simulink model "Trajectory_Tracking_Car_FL_MPC"  (R2024b)
settings: Solver=FixedStepAuto  StartTime=0.0  StopTime=63  FixedStep=Ts  RelTol=1e-3
values from neighbouring files (symbols this model uses):
  alpha = 3    [Setup_Trajectory_FL_MPC.m]    (also in Setup_trajectory_Backstepping.m; Setup_trajectory_NL_MPC.m)
  beta = 1.7    [Setup_Trajectory_FL_MPC.m]    (also in Setup_trajectory_Backstepping.m; Setup_trajectory_NL_MPC.m)
  Delta = 0.35    [Setup_Trajectory_FL_MPC.m]    (also in Setup_trajectory_NL_MPC.m)
  g_N = P_N.b    [Setup_Trajectory_FL_MPC.m]
  H_N = P_N.A    [Setup_Trajectory_FL_MPC.m]
  H_w = H_w/g_w(1)    [Setup_Trajectory_FL_MPC.m]    (also in Setup_trajectory_NL_MPC.m)
  Linv = linsolve(L,eye(size(L)),struct('LT',true))    [Setup_Trajectory_FL_MPC.m]
  N = 10    [Setup_Trajectory_FL_MPC.m]    (also in Setup_trajectory_Backstepping.m; Setup_trajectory_NL_MPC.m = 5)
  q0 = [x0;y0;theta0;phi0]    [Setup_Trajectory_FL_MPC.m]    (also in Setup_trajectory_Backstepping.m; Setup_trajectory_NL_MPC.m)
  qu = 0.00001    (= 1e-05)    [Setup_Trajectory_FL_MPC.m]    (also in Setup_trajectory_NL_MPC.m = 0.0001)
  qz = 10    [Setup_Trajectory_FL_MPC.m]    (also in Setup_trajectory_NL_MPC.m = 1)
  thetar = unwrap(atan2(ydr./v1r,xdr./v1r))    [Setup_Trajectory_FL_MPC.m]    (also in Setup_trajectory_Backstepping.m; Setup_trajectory_NL_MPC.m)
  Ts = 0.01    [Setup_Trajectory_FL_MPC.m]    (also in Setup_trajectory_Backstepping.m; Setup_trajectory_NL_MPC.m = 0.1)
  v1max = 2    [Setup_Trajectory_FL_MPC.m]    (also in Setup_trajectory_Backstepping.m; Setup_trajectory_NL_MPC.m)
  v2max = 2    [Setup_Trajectory_FL_MPC.m]    (also in Setup_trajectory_Backstepping.m = 10; Setup_trajectory_NL_MPC.m)
settings Model: Creator=cricr  LastModifiedBy=tirio
settings SolverCC: AlgebraicLoopSolver=TrustRegion
settings DataIOCC: ReturnWorkspaceOutputs=off
settings OptimizationCC: ReuseModelBlockBuffer=off
settings DebuggingCC: UnconnectedInputMsg=warning  UnconnectedOutputMsg=warning  UnconnectedLineMsg=warning  ArithmeticOperatorsInVariantConditions=warning
settings ModelReferenceCC: EnableRefExpFcnMdlSchedulingChecks=on
settings SFSimCC: SimUseLocalCustomCode=off  CustomCodeUndefinedFunction=UseInterfaceOnly
settings RTWCC: RTWUseLocalCustomCode=off  GPUComputeCapability=3.5

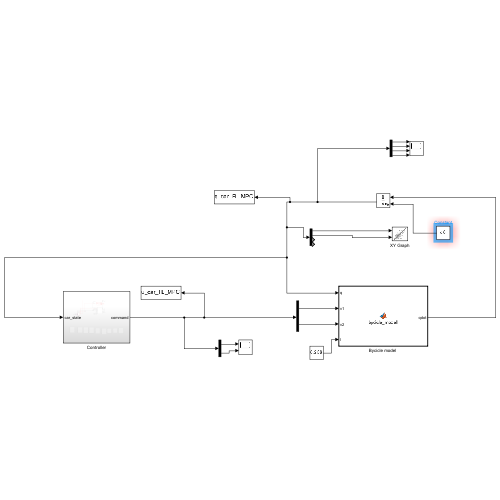
[thumbnail: Simulink's stored preview of the top-level diagram]
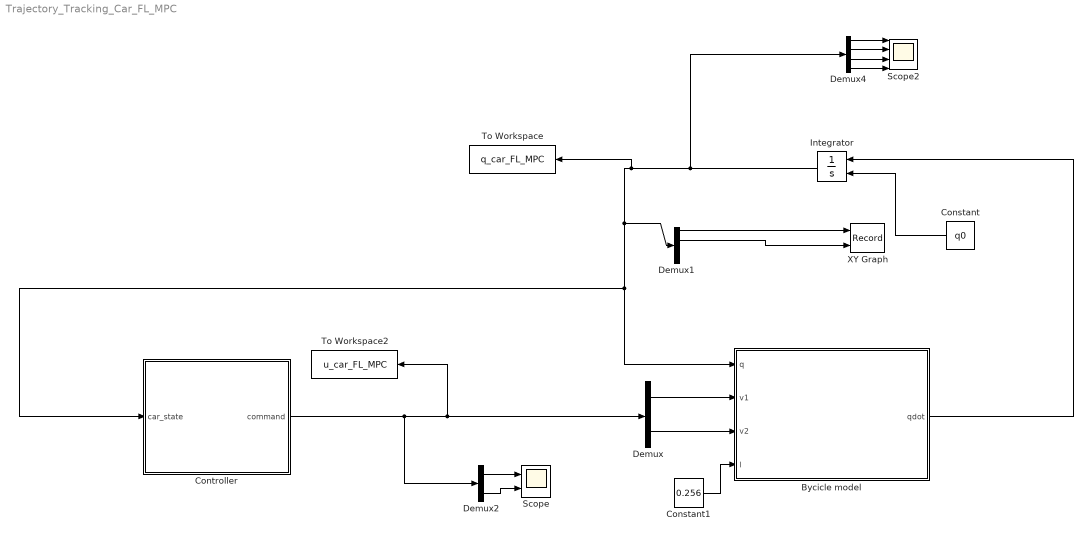
== system Trajectory_Tracking_Car_FL_MPC ==
  "Bycicle model " : MATLAB Function  TreatAsAtomicUnit=on
  Constant : Constant  Value=q0
  Constant1 : Constant  Value=0.256
  Controller : Subsystem
  Demux : Demux  Outputs=2
  Demux1 : Demux
  Demux2 : Demux  Outputs=2
  Demux4 : Demux
  Integrator : Integrator  InitialConditionSource=external
  Scope : Scope  NumInputPorts=2
  Scope2 : Scope  NumInputPorts=4
  To Workspace : ToWorkspace  VariableName=q_car_FL_MPC  SaveFormat=Timeseries  SampleTime=-1
  To Workspace2 : ToWorkspace  VariableName=u_car_FL_MPC  SaveFormat=Timeseries  SampleTime=-1
  XY Graph : Record  FileSettingsInternal="{\"entries\":[{\"content\":{\"excelSettings\":{\"content\":{},\"type\":\"Streamout.ExcelSettings\"}},\"type\":\"Streamout.FileSettingStorage\",\"uuid\":\"\"}],\"packageUris\":[\"http:\\/\\/schema.mathworks.com\\/mf0\\/streamout_blocks\\/R2020a\"],\"version\":\"1.0\"}"  Layout=[1 1]  SignalsInternal="{\"entries\":[{\"content\":{\"signals\":[{\"content\":{\"blockPath\":[],\"dimensions\":[1],\"domain\":\"\",\"lineColor\":\"#77ac30\",\"port\":1,\"signalID\":1,\"signalName\":\"Demux1:1\"},\"type\":\"RecordBlkView.Signal\",\"uuid\":\"\"},{\"content\":{\"blockPath\":[],\"dimensions\":[1],\"domain\":\"\",\"lineColor\":\"#4dbeee\",\"port\":2,\"signalID\":2,\"signalName\":\"Demux1:2\"},\"type\":\"RecordBlkView.Signal\",\"uuid\":\"\"}]},\"type\":\"RecordBlkView.InputSignals\",\"uuid\":\"\"}],\"packageUris\":[\"http:\\/\\/schema.mathworks.com\\/mf0\\/streamout_blocks\\/R2020a\"],\"version\":\"1.0\"}"  VisualizationBindings="{\"xyplotplugin\":{\"info\":[{\"series\":[],\"subplotID\":1}]}}"  CompatibilityTag=XY
  wires:
  "Bycicle model "/1(qdot) -> Integrator/1
  Constant1/1 -> "Bycicle model "/4(l)
  Demux/1 -> "Bycicle model "/2(v1)
  Demux/2 -> "Bycicle model "/3(v2)
  Demux1/1 -> XY Graph/1
  Demux1/2 -> XY Graph/2
  Demux4/4 -> Scope2/4
  Demux4/2 -> Scope2/2
  Demux4/3 -> Scope2/3
  Demux4/1 -> Scope2/1
  Constant/1 -> Integrator/2
  Integrator/1 -> Demux4/1, To Workspace/1, Controller/1(car_state), "Bycicle model "/1(q), Demux1/1
  Demux2/2 -> Scope/2
  Demux2/1 -> Scope/1
  Controller/1(command) -> Demux2/1, To Workspace2/1, Demux/1

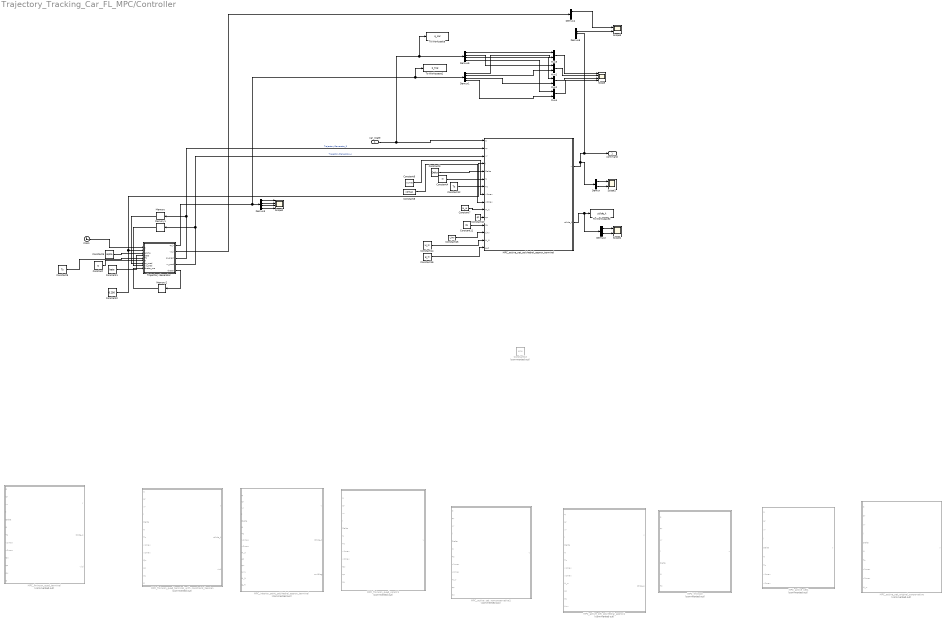
== system Trajectory_Tracking_Car_FL_MPC/Controller ==
  car_state : Inport
  Clock : Clock
  Constant : Constant  Value=N
  Constant1 : Constant  Value=beta
  Constant10 : Constant  Value=qz
  Constant11 : Constant  Value=qu
  Constant12 : Constant  Value=Ts
  Constant13 : Constant  Commented=on  Value=Linv
  Constant14 : Constant  Value=H_N
  Constant15 : Constant  Value=Linv
  Constant16 : Constant  Value=g_N
  Constant2 : Constant  Value=0.256
  Constant3 : Constant  Value=Delta
  Constant4 : Constant  Value=N
  Constant5 : Constant  Value=alpha
  Constant6 : Constant  Value=v1max
  Constant7 : Constant  Value=H_w
  Constant8 : Constant  Value=v2max
  Constant9 : Constant  Value=Ts
  Demux{,2,4,6} (4 alike) : Demux  Outputs=2
  Demux1 : Demux
  Demux3 : Demux
  Demux5 : Demux
  MPC_active_set1 : MATLAB Function  Commented=on  TreatAsAtomicUnit=on
  MPC_active_set_nonconservative1 : MATLAB Function  Commented=on  TreatAsAtomicUnit=on
  MPC_active_set_original_conservative : MATLAB Function  Commented=on  TreatAsAtomicUnit=on
  MPC_active_set_polyhedral_approx1 : MATLAB Function  Commented=on  TreatAsAtomicUnit=on
  MPC_active_set_polyhedral_approx_terminal : MATLAB Function  TreatAsAtomicUnit=on
  MPC_fmincon : MATLAB Function  Commented=on  TreatAsAtomicUnit=on
  MPC_fmincon_quad_constr1 : MATLAB Function  Commented=on  TreatAsAtomicUnit=on
  MPC_fmincon_quad_terminal : MATLAB Function  Commented=on  TreatAsAtomicUnit=on
  MPC_fmincon_quad_terminal_with_constraint_hessian : MATLAB Function  Commented=on  TreatAsAtomicUnit=on
  MPC_interior_point_polyhedral_approx_terminal : MATLAB Function  Commented=on  TreatAsAtomicUnit=on
  Memory : Memory  InitialCondition=zeros(4,N)
  Memory1 : Memory  InitialCondition=zeros(2,N)
  Memory2 : Memory  InitialCondition=thetar(1)
  Mux{1..4} (4 alike) : Mux  Inputs=2
  Scope : Scope  NumInputPorts=4
  Scope1 : Scope  NumInputPorts=2
  Scope2 : Scope  NumInputPorts=4
  Scope3 : Scope  NumInputPorts=2
  Scope4 : Scope  NumInputPorts=2
  To Workspace : ToWorkspace  VariableName=q_car  SaveFormat=Timeseries  SampleTime=-1
  To Workspace1 : ToWorkspace  VariableName=q_traj  SaveFormat=Timeseries  SampleTime=-1
  To Workspace2 : ToWorkspace  VariableName=ztilde_k  SaveFormat=Timeseries  SampleTime=-1
  Trajectory Generator : MATLAB Function  TreatAsAtomicUnit=on
  command : Outport
  wires:
  Demux5/2 -> Mux1/1
  Constant6/1 -> MPC_active_set_polyhedral_approx_terminal/8(v1max)
  Demux6/1 -> Scope3/2
  Demux5/4 -> Mux4/1
  Mux2/1 -> Scope/3
  Mux3/1 -> Scope/1
  Demux3/1 -> Scope2/1
  Demux4/1 -> Scope3/1
  Demux1/3 -> Mux2/2
  Mux1/1 -> Scope/2
  Demux1/4 -> Mux4/2
  Mux4/1 -> Scope/4
  Constant7/1 -> MPC_active_set_polyhedral_approx_terminal/10(H_w)
  Demux3/2 -> Scope2/2
  Demux5/1 -> Mux3/1
  Demux3/4 -> Scope2/4
  car_state/1 -> To Workspace/1, Demux5/1, MPC_active_set_polyhedral_approx_terminal/1(q)
  Constant8/1 -> MPC_active_set_polyhedral_approx_terminal/9(v2max)
  Demux1/1 -> Mux3/2
  MPC_active_set_polyhedral_approx_terminal/1(v) -> Demux/1, Demux6/1, command/1
  Demux1/2 -> Mux1/2
  Demux5/3 -> Mux2/1
  Demux3/3 -> Scope2/3
  Memory1/1 -> Trajectory Generator/8("vr_pred ")
  Memory/1 -> Trajectory Generator/7("qr_pred ")
  Trajectory Generator/3(qr_pred) -> MPC_active_set_polyhedral_approx_terminal/2(qr), Memory/1  "TrajectoryGenerator_3"
  Constant/1 -> Trajectory Generator/6(N)
  Trajectory Generator/4(vr_pred) -> MPC_active_set_polyhedral_approx_terminal/3(vr), Memory1/1  "TrajectoryGenerator_4"
  Constant1/1 -> Trajectory Generator/4(beta)
  Constant2/1 -> MPC_active_set_polyhedral_approx_terminal/4(l), Trajectory Generator/2(l)
  Constant9/1 -> Trajectory Generator/5(Ts)
  Constant5/1 -> Trajectory Generator/3(alpha)
  Trajectory Generator/5(thetar) -> Memory2/1
  Clock/1 -> Trajectory Generator/1(t)
  Memory2/1 -> Trajectory Generator/9(thetar_pre)
  Trajectory Generator/2(vr_k) -> Demux4/1
  Trajectory Generator/1(qr_k) -> To Workspace1/1, Demux1/1, Demux3/1
  Constant11/1 -> MPC_active_set_polyhedral_approx_terminal/12(qu)
  Constant3/1 -> MPC_active_set_polyhedral_approx_terminal/5(Delta)
  Constant12/1 -> MPC_active_set_polyhedral_approx_terminal/7(Ts)
  Constant14/1 -> MPC_active_set_polyhedral_approx_terminal/14(H_N)
  Demux/1 -> Scope1/1
  Demux/2 -> Scope1/2
  Constant15/1 -> MPC_active_set_polyhedral_approx_terminal/13(Linv)
  Demux2/2 -> Scope4/2
  Demux2/1 -> Scope4/1
  MPC_active_set_polyhedral_approx_terminal/2(ztilde_k) -> Demux2/1, To Workspace2/1
  Constant16/1 -> MPC_active_set_polyhedral_approx_terminal/15(g_N)
  Constant4/1 -> MPC_active_set_polyhedral_approx_terminal/6(N)
  Constant10/1 -> MPC_active_set_polyhedral_approx_terminal/11(qz)

== matlab function Trajectory_Tracking_Car_FL_MPC/Controller/Trajectory Generator ==
  data: t input; qr_k output; vr_k output; l input; alpha input; beta input; Ts input; qr_pred output size=[4 N]; vr_pred output size=[2 N]; N input; qr_pred input; vr_pred input; thetar_pre input; thetar output
function [qr_k,vr_k,qr_pred, vr_pred,thetar] = Trajectory(t,l,alpha,beta,Ts,N,qr_pred,vr_pred,thetar_pre)




xr=alpha*sin(t/beta);
yr=alpha*sin(t/(2*beta));

xdr=alpha*cos(t/beta)*(1/(beta));
ydr=alpha*cos(t/(2*beta))*(1/(2*beta));


xddr=-alpha*sin(t/beta)*(1/(beta))^2;
yddr=-alpha*sin(t/(2*beta))*(1/(2*beta))^2;

xdddr=-alpha*cos(t/beta)*(1/(beta))^3;
ydddr=-alpha*cos(t/(2*beta))*(1/(2*beta))^3;

%Driving velocity reference
v1r=sqrt(xdr^2+ydr^2); %Linear velocity of the trajectory


thetar=atan2(ydr/v1r,xdr/v1r);

theta=[thetar_pre thetar];

theta=unwrap(theta);
thetar=theta(2);


%Steering angle reference
phir=atan(l*(yddr*xdr-xddr*ydr)/v1r^3);

%Steering velocity reference
v2r=l*v1r*((ydddr*xdr-xdddr*ydr)*v1r^2-3*(yddr*xdr-xddr*ydr)*(xdr*xddr+ydr*yddr))/(v1r^6+l^2*(yddr*xdr-xddr*ydr)^2);


qr_k=[xr;yr;thetar;phir];
vr_k=[v1r;v2r];


for i=1:N
    t=t+(i-1)*Ts;
    xr=alpha*sin(t/beta);
    yr=alpha*sin(t/(2*beta));

    xdr=alpha*cos(t/beta)*(1/(beta));
    ydr=alpha*cos(t/(2*beta))*(1/(2*beta));


    xddr=-alpha*sin(t/beta)*(1/(beta))^2;
    yddr=-alpha*sin(t/(2*beta))*(1/(2*beta))^2;

    xdddr=-alpha*cos(t/beta)*(1/(beta))^3;
    ydddr=-alpha*cos(t/(2*beta))*(1/(2*beta))^3;



    %Driving velocity reference
    v1r=sqrt(xdr^2+ydr^2); %Linear velocity of the trajectory

    

    thetar=atan2(ydr/v1r,xdr/v1r);

    if i==1
        theta=[thetar_pre thetar];
        theta=unwrap(theta);
        thetar=theta(2);
        thetar_pre=thetar;

    else
       
        theta=[thetar_pre thetar];
        theta=unwrap(theta);
        thetar=theta(2);


    end


    %Steering angle reference
    phir=atan(l*(yddr*xdr-xddr*ydr)/v1r^3);

    %Steering velocity reference
    v2r=l*v1r*((ydddr*xdr-xdddr*ydr)*v1r^2-3*(yddr*xdr-xddr*ydr)*(xdr*xddr+ydr*yddr))/(v1r^6+l^2*(yddr*xdr-xddr*ydr)^2);



    %Nonlinear model reference state
    qr_pred(:,i)=[xr;yr;thetar;phir];
    vr_pred(:,i)=[v1r;v2r];

end

 qr_pred(3,:)= unwrap(qr_pred(3,:));

== matlab function Trajectory_Tracking_Car_FL_MPC/Controller/MPC_active_set_nonconservative1 ==
  data: q input; v output; qr input; vr input; l input; Delta input; N input; Ts input; v1max input; v2max input; H_w input; qz input; qu input
function v = MPC_analytical(q,qr,vr,l,Delta,N,Ts,v1max,v2max,H_w,qz,qu)


x=q(1); y=q(2); theta=q(3); phi=q(4);

%Feedback linearized system state
z_k=[x+l*cos(theta)+Delta*cos(phi+theta);
    y+l*sin(theta)+Delta*sin(phi+theta)];


Wr=zeros(2*N,1);
R=zeros(2*N,1);



for i=1:N
    xr=qr(1,i); yr=qr(2,i); thetar=qr(3,i); phir=qr(4,i);
    v1r=vr(1,i); v2r=vr(2,i);

    %Feedback linearized system reference at time k+i
    zr_k=[xr+l*cos(thetar)+Delta*cos(phir+thetar);
        yr+l*sin(thetar)+Delta*sin(phir+thetar)];

    R(2*i-1:2*i,1)=zr_k;

    %Feedback Linearization reference transformation
    T_FL_r=[cos(thetar)-tan(phir)*(sin(thetar)+Delta*sin(thetar+phir)/l) -Delta*sin(thetar+phir);
        sin(thetar)+tan(phir)*(cos(thetar)+Delta*cos(thetar+phir)/l) Delta*cos(thetar+phir)];

    ur_k=T_FL_r*[v1r;v2r];

    Wr(2*i-1:2*i,1)=ur_k;


end


%Feedback Linearization state transformation
T_FL=[cos(theta)-tan(phi)*(sin(theta)+Delta*sin(theta+phi)/l) -Delta*sin(theta+phi);
    sin(theta)+tan(phi)*(cos(theta)+Delta*cos(theta+phi)/l) Delta*cos(theta+phi)];





Phi=repmat(eye(2),N,1);
Theta=Ts*repmat(eye(2),N);
Theta=tril(Theta);
Qhat=qz*eye(2*N);
Rhat=qu*eye(2*N);







H_obj=Theta'*Qhat*Theta+Rhat;
f_obj=Theta'*Qhat*Phi*z_k-Theta'*Qhat*Theta*Wr-Theta'*Qhat*R;
% 
% T=[-1 0; 0 -1; 1 0; 0 1];
% Hk=T/T_FL;
% g=[v1max;v2max;v1max;v2max];
% 
% H_constr=zeros(4,2*N);
% H_constr(1:4,1:2)=Hk;

% for i=1:N-1
%     
%     H_constr(4+(i-1)*Nc+1:4+(i-1)*Nc+Nc,2*i+1:2*i+2)=H_w;
% 
% 
% end


% 
% g_constr=zeros(size(H_constr,1),1);
% g_constr(1:4)=g;
% 
% 
% 

% options = optimoptions('quadprog','Algorithm','active-set');
% usol =  quadprog(H_obj,f_obj,H_constr,g_constr,[],[],[],[],zeros(2*N,1),options);




% opt.MaxIterations = 100;
% opt.ConstraintTolerance = 1.0e-6;
% % opt.OptimalityTolerance = 1.0e-6;
% 
% opt = mpcInteriorPointOptions;
% usol=mpcInteriorPointSolver(H_obj,f_obj,H_constr,g_constr,zeros(0,2*N),zeros(0,1),zeros(2*N,1),opt);
% % 

% opt.UseHessianAsInput = true;
% iA0 = false(size(g_constr));
% usol=mpcActiveSetSolver(H_obj,f_obj,H_constr,g_constr,zeros(0,2*N),zeros(0,1),iA0,opt);



usol=-H_obj\f_obj;

uk=usol(1:2);



v=T_FL\uk;

== matlab function Trajectory_Tracking_Car_FL_MPC/Controller/MPC_active_set_polyhedral_approx_terminal ==
  data: q input; v output; qr input; vr input; l input; Delta input; N input; Ts input; v1max input; v2max input; H_w input; qz input; qu input; Linv input; H_N input; ztilde_k output; g_N input
function [v,ztilde_k] = MPC_active_set_polyhedral_approx(q,qr,vr,l,Delta,N,Ts,v1max,v2max,H_w,qz,qu,Linv,H_N,g_N)


x=q(1); y=q(2); theta=q(3); phi=q(4);

%Feedback linearized system state
z_k=[x+l*cos(theta)+Delta*cos(phi+theta);
     y+l*sin(theta)+Delta*sin(phi+theta)];


xr=qr(1,1); yr=qr(2,1); thetar=qr(3,1); phir=qr(4,1);
%Feedback linearized system reference at time k+i
zr_k=[xr+l*cos(thetar)+Delta*cos(phir+thetar);
      yr+l*sin(thetar)+Delta*sin(phir+thetar)];

ztilde_k=z_k-zr_k;


Wr=zeros(2*N,1);
% R=zeros(2*N,1);



for i=1:N
    thetar=qr(3,i); phir=qr(4,i);
    v1r=vr(1,i); v2r=vr(2,i);

    %     R(2*i-1:2*i,1)=zr_k;

    %Feedback Linearization reference transformation
    T_FL_r=[cos(thetar)-tan(phir)*(sin(thetar)+Delta*sin(thetar+phir)/l) -Delta*sin(thetar+phir);
        sin(thetar)+tan(phir)*(cos(thetar)+Delta*cos(thetar+phir)/l) Delta*cos(thetar+phir)];

    ur_k=T_FL_r*[v1r;v2r];

    Wr(2*i-1:2*i,1)=ur_k;


end


%Feedback Linearization state transformation
T_FL=[cos(theta)-tan(phi)*(sin(theta)+Delta*sin(theta+phi)/l) -Delta*sin(theta+phi);
    sin(theta)+tan(phi)*(cos(theta)+Delta*cos(theta+phi)/l) Delta*cos(theta+phi)];





Phi=repmat(eye(2),N,1);
Theta=Ts*repmat(eye(2),N);
Theta=tril(Theta);
Qhat=qz*eye(2*N);
Rhat=qu*eye(2*N);
Theta_N=Theta(2*N-1:2*N,:);
Phi_N=eye(2);


% H_obj=Theta'*Qhat*Theta+Rhat;
f_obj=Theta'*Qhat*Phi*ztilde_k-Theta'*Qhat*Theta*Wr-Rhat*Wr;

T=[-1 0; 0 -1; 1 0; 0 1];
Hk=T/T_FL;
g=[v1max;v2max;v1max;v2max];



Nc1=size(H_w,1);
H_constr1=zeros(4+Nc1*(N-1),2*N);
H_constr1(1:4,1:2)=Hk;

for i=1:N-1
    
    H_constr1(4+(i-1)*Nc1+1:4+(i-1)*Nc1+Nc1,2*i+1:2*i+2)=H_w;


end

g_constr1=ones(size(H_constr1,1),1);
g_constr1(1:4)=g;



H_constr2=H_N*Theta_N;
g_constr2=g_N-H_N*Phi_N*ztilde_k;

H_constr=[H_constr1;H_constr2];
g_constr=[g_constr1;g_constr2];


% options = optimoptions('quadprog','Algorithm','active-set');
% usol =  quadprog(H_obj,f_obj,H_constr,g_constr,[],[],[],[],zeros(2*N,1),options);




% opt = mpcInteriorPointOptions;
% 
% opt.MaxIterations = 100;
% opt.ConstraintTolerance = 1.0e-6;
% opt.OptimalityTolerance = 1.0e-6;
% 
% usol=mpcInteriorPointSolver(H_obj,f_obj,H_constr,g_constr,zeros(0,2*N),zeros(0,1),zeros(2*N,1),opt);

%
opt = mpcActiveSetOptions;
% opt.UseHessianAsInput = true;
opt.UseHessianAsInput = false;
opt.MaxIterations = 50;
opt.ConstraintTolerance = 1.0e-6;
opt.OptimalityTolerance = 1.0e-6;

iA0 = false(size(g_constr));
% usol=mpcActiveSetSolver(H_obj,f_obj,H_constr,g_constr,zeros(0,2*N),zeros(0,1),iA0,opt);
usol=mpcActiveSetSolver(Linv,f_obj,H_constr,g_constr,zeros(0,2*N),zeros(0,1),iA0,opt);


check=H_constr2*usol<=g_constr2;
viol=true;
for i=1:length(check)
    viol=viol&check(i);
end

viol



disp('Next step')
uk=usol(1:2);



v=T_FL\uk;

== matlab function Trajectory_Tracking_Car_FL_MPC/Controller/MPC_active_set_polyhedral_approx1 ==
  data: q input; v output; qr input; vr input; l input; Delta input; N input; Ts input; v1max input; v2max input; H_w input; qz input; qu input; Linv input; ztilde_k output
function [v,ztilde_k]= MPC_active_set_polyhedral_approx(q,qr,vr,l,Delta,N,Ts,v1max,v2max,H_w,qz,qu,Linv)


x=q(1); y=q(2); theta=q(3); phi=q(4);

%Feedback linearized system state
z_k=[x+l*cos(theta)+Delta*cos(phi+theta);
     y+l*sin(theta)+Delta*sin(phi+theta)];


xr=qr(1,1); yr=qr(2,1); thetar=qr(3,1); phir=qr(4,1);
%Feedback linearized system reference at time k+i
zr_k=[xr+l*cos(thetar)+Delta*cos(phir+thetar);
      yr+l*sin(thetar)+Delta*sin(phir+thetar)];

ztilde_k=z_k-zr_k;


Wr=zeros(2*N,1);
% R=zeros(2*N,1);



for i=1:N
    thetar=qr(3,i); phir=qr(4,i);
    v1r=vr(1,i); v2r=vr(2,i);

    %     R(2*i-1:2*i,1)=zr_k;

    %Feedback Linearization reference transformation
    T_FL_r=[cos(thetar)-tan(phir)*(sin(thetar)+Delta*sin(thetar+phir)/l) -Delta*sin(thetar+phir);
        sin(thetar)+tan(phir)*(cos(thetar)+Delta*cos(thetar+phir)/l) Delta*cos(thetar+phir)];

    ur_k=T_FL_r*[v1r;v2r];

    Wr(2*i-1:2*i,1)=ur_k;


end


%Feedback Linearization state transformation
T_FL=[cos(theta)-tan(phi)*(sin(theta)+Delta*sin(theta+phi)/l) -Delta*sin(theta+phi);
    sin(theta)+tan(phi)*(cos(theta)+Delta*cos(theta+phi)/l) Delta*cos(theta+phi)];





Phi=repmat(eye(2),N,1);
Theta=Ts*repmat(eye(2),N);
Theta=tril(Theta);
Qhat=qz*eye(2*N);
Rhat=qu*eye(2*N);


% H_obj=Theta'*Qhat*Theta+Rhat;
f_obj=Theta'*Qhat*Phi*ztilde_k-Theta'*Qhat*Theta*Wr-Rhat*Wr;

T=[-1 0; 0 -1; 1 0; 0 1];
Hk=T/T_FL;
g=[v1max;v2max;v1max;v2max];



Nc=size(H_w,1);
H_constr=zeros(4+Nc*(N-1),2*N);
H_constr(1:4,1:2)=Hk;

for i=1:N-1
    
    H_constr(4+(i-1)*Nc+1:4+(i-1)*Nc+Nc,2*i+1:2*i+2)=H_w;


end

g_constr=ones(size(H_constr,1),1);
g_constr(1:4)=g;





% options = optimoptions('quadprog','Algorithm','active-set');
% usol =  quadprog(H_obj,f_obj,H_constr,g_constr,[],[],[],[],zeros(2*N,1),options);




% opt = mpcInteriorPointOptions;
% 
% opt.MaxIterations = 100;
% opt.ConstraintTolerance = 1.0e-6;
% opt.OptimalityTolerance = 1.0e-6;
% 
% usol=mpcInteriorPointSolver(H_obj,f_obj,H_constr,g_constr,zeros(0,2*N),zeros(0,1),zeros(2*N,1),opt);

%
opt = mpcActiveSetOptions;
% opt.UseHessianAsInput = true;
opt.UseHessianAsInput = false;
opt.MaxIterations = 50;
opt.ConstraintTolerance = 1.0e-6;
opt.OptimalityTolerance = 1.0e-6;

iA0 = false(size(g_constr));
% usol=mpcActiveSetSolver(H_obj,f_obj,H_constr,g_constr,zeros(0,2*N),zeros(0,1),iA0,opt);
usol=mpcActiveSetSolver(Linv,f_obj,H_constr,g_constr,zeros(0,2*N),zeros(0,1),iA0,opt);

uk=usol(1:2);



v=T_FL\uk;

== matlab function Trajectory_Tracking_Car_FL_MPC/Controller/MPC_interior_point_polyhedral_approx_terminal ==
  data: q input; v output; qr input; vr input; l input; Delta input; N input; Ts input; v1max input; v2max input; H_w input; qz input; qu input; Linv input; H_N input; ztilde_k output; g_N input; exitflag output
function [v,ztilde_k,exitflag] = MPC_interior_point_polyhedral_approx(q,qr,vr,l,Delta,N,Ts,v1max,v2max,H_w,qz,qu,Linv,H_N,g_N)


x=q(1); y=q(2); theta=q(3); phi=q(4);

%Feedback linearized system state
z_k=[x+l*cos(theta)+Delta*cos(phi+theta);
     y+l*sin(theta)+Delta*sin(phi+theta)];


xr=qr(1,1); yr=qr(2,1); thetar=qr(3,1); phir=qr(4,1);
%Feedback linearized system reference at time k+i
zr_k=[xr+l*cos(thetar)+Delta*cos(phir+thetar);
      yr+l*sin(thetar)+Delta*sin(phir+thetar)];

ztilde_k=z_k-zr_k;


Wr=zeros(2*N,1);
% R=zeros(2*N,1);



for i=1:N
    thetar=qr(3,i); phir=qr(4,i);
    v1r=vr(1,i); v2r=vr(2,i);

    %     R(2*i-1:2*i,1)=zr_k;

    %Feedback Linearization reference transformation
    T_FL_r=[cos(thetar)-tan(phir)*(sin(thetar)+Delta*sin(thetar+phir)/l) -Delta*sin(thetar+phir);
        sin(thetar)+tan(phir)*(cos(thetar)+Delta*cos(thetar+phir)/l) Delta*cos(thetar+phir)];

    ur_k=T_FL_r*[v1r;v2r];

    Wr(2*i-1:2*i,1)=ur_k;


end


%Feedback Linearization state transformation
T_FL=[cos(theta)-tan(phi)*(sin(theta)+Delta*sin(theta+phi)/l) -Delta*sin(theta+phi);
    sin(theta)+tan(phi)*(cos(theta)+Delta*cos(theta+phi)/l) Delta*cos(theta+phi)];





Phi=repmat(eye(2),N,1);
Theta=Ts*repmat(eye(2),N);
Theta=tril(Theta);
Qhat=qz*eye(2*N);
Rhat=qu*eye(2*N);
Theta_N=Theta(2*N-1:2*N,:);
Phi_N=eye(2);


H_obj=Theta'*Qhat*Theta+Rhat;
f_obj=Theta'*Qhat*Phi*ztilde_k-Theta'*Qhat*Theta*Wr-Rhat*Wr;

T=[-1 0; 0 -1; 1 0; 0 1];
Hk=T/T_FL;
g=[v1max;v2max;v1max;v2max];



Nc1=size(H_w,1);
H_constr1=zeros(4+Nc1*(N-1),2*N);
H_constr1(1:4,1:2)=Hk;

for i=1:N-1
    
    H_constr1(4+(i-1)*Nc1+1:4+(i-1)*Nc1+Nc1,2*i+1:2*i+2)=H_w;


end

g_constr1=ones(size(H_constr1,1),1);
g_constr1(1:4)=g;



H_constr2=H_N*Theta_N;
g_constr2=g_N-H_N*Phi_N*ztilde_k;

H_constr=[H_constr1;H_constr2];
g_constr=[g_constr1;g_constr2];


% options = optimoptions('quadprog','Algorithm','active-set');
% usol =  quadprog(H_obj,f_obj,H_constr,g_constr,[],[],[],[],zeros(2*N,1),options);




opt = mpcInteriorPointOptions;

opt.MaxIterations = 100;
opt.ConstraintTolerance = 1.0e-6;
opt.OptimalityTolerance = 1.0e-6;

[usol, exitflag ]=mpcInteriorPointSolver(H_obj,f_obj,H_constr,g_constr,zeros(0,2*N),zeros(0,1),zeros(2*N,1),opt);

% %
% opt = mpcActiveSetOptions;
% % opt.UseHessianAsInput = true;
% opt.UseHessianAsInput = false;
% opt.MaxIterations = 50;
% opt.ConstraintTolerance = 1.0e-6;
% opt.OptimalityTolerance = 1.0e-6;
% 
% iA0 = false(size(g_constr));
% % usol=mpcActiveSetSolver(H_obj,f_obj,H_constr,g_constr,zeros(0,2*N),zeros(0,1),iA0,opt);
% usol=mpcActiveSetSolver(Linv,f_obj,H_constr,g_constr,zeros(0,2*N),zeros(0,1),iA0,opt);


check=H_constr*usol<=g_constr;
viol=true;
for i=1:length(check)
    viol=viol&check(i);
end

viol



disp('Next step')
uk=usol(1:2);



v=T_FL\uk;

== matlab function Trajectory_Tracking_Car_FL_MPC/Controller/MPC_fmincon_quad_constr1 ==
  data: q input; v output; qr input; vr input; l input; Delta input; N input; Ts input; v1max input; v2max input; Qu input; qz input; qu input
function v = MPC_quad_constr(q,qr,vr,l,Delta,N,Ts,v1max,v2max,Qu,qz,qu)


x=q(1); y=q(2); theta=q(3); phi=q(4);

%Feedback linearized system state
z_k=[x+l*cos(theta)+Delta*cos(phi+theta);
    y+l*sin(theta)+Delta*sin(phi+theta)];



xr=qr(1,1); yr=qr(2,1); thetar=qr(3,1); phir=qr(4,1);
%Feedback linearized system reference at time k+i
zr_k=[xr+l*cos(thetar)+Delta*cos(phir+thetar);
      yr+l*sin(thetar)+Delta*sin(phir+thetar)];

ztilde_k=z_k-zr_k;

Wr=zeros(2*N,1);


for i=1:N
    thetar=qr(3,i); phir=qr(4,i);
    v1r=vr(1,i); v2r=vr(2,i);

    %     R(2*i-1:2*i,1)=zr_k;

    %Feedback Linearization reference transformation
    T_FL_r=[cos(thetar)-tan(phir)*(sin(thetar)+Delta*sin(thetar+phir)/l) -Delta*sin(thetar+phir);
        sin(thetar)+tan(phir)*(cos(thetar)+Delta*cos(thetar+phir)/l) Delta*cos(thetar+phir)];

    ur_k=T_FL_r*[v1r;v2r];

    Wr(2*i-1:2*i,1)=ur_k;
end


%Feedback Linearization state transformation
T_FL=[cos(theta)-tan(phi)*(sin(theta)+Delta*sin(theta+phi)/l) -Delta*sin(theta+phi);
    sin(theta)+tan(phi)*(cos(theta)+Delta*cos(theta+phi)/l) Delta*cos(theta+phi)];





Phi=repmat(eye(2),N,1);
Theta=Ts*repmat(eye(2),N);
Theta=tril(Theta);
Qhat=qz*eye(2*N);
Rhat=qu*eye(2*N);




H_obj=Theta'*Qhat*Theta+Rhat;
f_obj=Theta'*Qhat*Phi*ztilde_k-Theta'*Qhat*Theta*Wr-Rhat*Wr;

T=[-1 0; 0 -1; 1 0; 0 1];
Hk=T/T_FL;
g=[v1max;v2max;v1max;v2max];











%obj_fun=@(W)(Phi*z_k+Theta*(W-Wr)-R)'*Qhat*(Phi*z_k+Theta*(W-Wr)-R)+W'*Rhat*W;

obj_fun=@(u)(u'*H_obj*u+f_obj'*u);

    function [c,ceq]=quad_constr(u,Hk,g,Qu,N)
        H_constr=zeros(4,2*N);
        H_constr(1:4,1:2)=Hk;

        g_constr=zeros(size(H_constr,1),1);
        g_constr(1:4)=g;

        c1=H_constr*u-g_constr;

        q_u=Qu(1,1);
        Qu_hat=zeros(2*N,2*N);

        for k=3:2*N
           Qu_hat(k,k)=q_u;
        end

        c2=u'*Qu_hat*u-1;

        

        c=[c1;c2];
        ceq=[];
    end



options=optimoptions('fmincon','Display','off','Algorithm','sqp');
usol = fmincon(obj_fun,zeros(N*2,1),[],[],[],[],[],[],@(u)quad_constr(u,Hk,g,Qu,N),options);



uk=usol(1:2);



v=T_FL\uk;


end

== matlab function Trajectory_Tracking_Car_FL_MPC/Controller/MPC_fmincon_quad_terminal ==
  data: q input; v output; qr input; vr input; l input; Delta input; N input; Ts input; v1max input; v2max input; Qu input; qz input; qu input; S input; ztilde_k output; viol output
function [v,ztilde_k,viol] = MPC_quad_terminal(q,qr,vr,l,Delta,N,Ts,v1max,v2max,Qu,qz,qu,S)


x=q(1); y=q(2); theta=q(3); phi=q(4);

%Feedback linearized system state
z_k=[x+l*cos(theta)+Delta*cos(phi+theta);
    y+l*sin(theta)+Delta*sin(phi+theta)];



xr=qr(1,1); yr=qr(2,1); thetar=qr(3,1); phir=qr(4,1);
%Feedback linearized system reference at time k+i
zr_k=[xr+l*cos(thetar)+Delta*cos(phir+thetar);
    yr+l*sin(thetar)+Delta*sin(phir+thetar)];

ztilde_k=z_k-zr_k;

Wr=zeros(2*N,1);


for i=1:N
    thetar=qr(3,i); phir=qr(4,i);
    v1r=vr(1,i); v2r=vr(2,i);

    %     R(2*i-1:2*i,1)=zr_k;

    %Feedback Linearization reference transformation
    T_FL_r=[cos(thetar)-tan(phir)*(sin(thetar)+Delta*sin(thetar+phir)/l) -Delta*sin(thetar+phir);
        sin(thetar)+tan(phir)*(cos(thetar)+Delta*cos(thetar+phir)/l) Delta*cos(thetar+phir)];

    ur_k=T_FL_r*[v1r;v2r];

    Wr(2*i-1:2*i,1)=ur_k;
end


%Feedback Linearization state transformation
T_FL=[cos(theta)-tan(phi)*(sin(theta)+Delta*sin(theta+phi)/l) -Delta*sin(theta+phi);
    sin(theta)+tan(phi)*(cos(theta)+Delta*cos(theta+phi)/l) Delta*cos(theta+phi)];





Phi=repmat(eye(2),N,1);
Theta=Ts*repmat(eye(2),N);
Theta=tril(Theta);
Qhat=qz*eye(2*N);
Rhat=qu*eye(2*N);
Theta_N=Theta(2*N-1:2*N,:);
Psi_N=eye(2);



H_obj=Theta'*Qhat*Theta+Rhat;
f_obj=Theta'*Qhat*Phi*ztilde_k-Theta'*Qhat*Theta*Wr-Rhat*Wr;

T=[-1 0; 0 -1; 1 0; 0 1];
Hk=T/T_FL;
g=[v1max;v2max;v1max;v2max];











%obj_fun=@(W)(Phi*z_k+Theta*(W-Wr)-R)'*Qhat*(Phi*z_k+Theta*(W-Wr)-R)+W'*Rhat*W;



    function [obj_fun,gradient]=objective_function(u,H_obj,f_obj)
        obj_fun=u'*H_obj*u+f_obj'*u;
        gradient=2*H_obj*u+f_obj;
    end

    function [c,ceq]=quad_constr(u,Hk,g,Qu,N,Theta_N,Psi_N,S,ztilde_k)
        H_constr=zeros(4,2*N);
        H_constr(1:4,1:2)=Hk;

        g_constr=zeros(size(H_constr,1),1);
        g_constr(1:4)=g;

        c1=H_constr*u-g_constr

        q_u=Qu(1,1);
        Qu_hat=zeros(2*N,2*N);

        for k=3:2*N
            Qu_hat(k,k)=q_u;
        end

        c2=u'*Qu_hat*u-1


        c3=u'*(Theta_N'*S*Theta_N)*u+2*ztilde_k'*Psi_N'*S*Theta_N*u-1+ztilde_k'*Psi_N'*S*Psi_N*ztilde_k

        c=[c1;c2;c3];
        ceq=[];
    end



options=optimoptions('fmincon','Display','off','Algorithm','sqp-legacy','SpecifyObjectiveGradient',true);
    [usol,fval,exitflag,output,lambda,grad,hessian] = fmincon(@(u)objective_function(u,H_obj,f_obj),zeros(N*2,1),[],[],[],[],[],[],@(u)quad_constr(u,Hk,g,Qu,N,Theta_N,Psi_N,S,ztilde_k),options);


viol=output.constrviolation;


uk=usol(1:2);



v=T_FL\uk;


end

== matlab function Trajectory_Tracking_Car_FL_MPC/Controller/MPC_fmincon_quad_terminal_with_constraint_hessian ==
  data: q input; v output; qr input; vr input; l input; Delta input; N input; Ts input; v1max input; v2max input; Qu input; qz input; qu input; S input; ztilde_k output; viol output
function [v,ztilde_k,viol] = MPC_quad_terminal(q,qr,vr,l,Delta,N,Ts,v1max,v2max,Qu,qz,qu,S)


x=q(1); y=q(2); theta=q(3); phi=q(4);

%Feedback linearized system state
z_k=[x+l*cos(theta)+Delta*cos(phi+theta);
    y+l*sin(theta)+Delta*sin(phi+theta)];



xr=qr(1,1); yr=qr(2,1); thetar=qr(3,1); phir=qr(4,1);
%Feedback linearized system reference at time k+i
zr_k=[xr+l*cos(thetar)+Delta*cos(phir+thetar);
    yr+l*sin(thetar)+Delta*sin(phir+thetar)];

ztilde_k=z_k-zr_k;

Wr=zeros(2*N,1);


for i=1:N
    thetar=qr(3,i); phir=qr(4,i);
    v1r=vr(1,i); v2r=vr(2,i);

    %     R(2*i-1:2*i,1)=zr_k;

    %Feedback Linearization reference transformation
    T_FL_r=[cos(thetar)-tan(phir)*(sin(thetar)+Delta*sin(thetar+phir)/l) -Delta*sin(thetar+phir);
        sin(thetar)+tan(phir)*(cos(thetar)+Delta*cos(thetar+phir)/l) Delta*cos(thetar+phir)];

    ur_k=T_FL_r*[v1r;v2r];

    Wr(2*i-1:2*i,1)=ur_k;
end


%Feedback Linearization state transformation
T_FL=[cos(theta)-tan(phi)*(sin(theta)+Delta*sin(theta+phi)/l) -Delta*sin(theta+phi);
    sin(theta)+tan(phi)*(cos(theta)+Delta*cos(theta+phi)/l) Delta*cos(theta+phi)];





Phi=repmat(eye(2),N,1);
Theta=Ts*repmat(eye(2),N);
Theta=tril(Theta);
Qhat=qz*eye(2*N);
Rhat=qu*eye(2*N);
Theta_N=Theta(2*N-1:2*N,:);
Psi_N=eye(2);



H_obj=Theta'*Qhat*Theta+Rhat;
f_obj=Theta'*Qhat*Phi*ztilde_k-Theta'*Qhat*Theta*Wr-Rhat*Wr;

T=[-1 0; 0 -1; 1 0; 0 1];
Hk=T/T_FL;
g=[v1max;v2max;v1max;v2max];











%obj_fun=@(W)(Phi*z_k+Theta*(W-Wr)-R)'*Qhat*(Phi*z_k+Theta*(W-Wr)-R)+W'*Rhat*W;



    function [obj_fun,gradient]=objective_function(u,H_obj,f_obj)
        obj_fun=u'*H_obj*u+f_obj'*u;
        gradient=2*H_obj*u+f_obj;
    end

    function [c,ceq,gradc,gradceq]=quad_constr(u,Hk,g,Qu,N,Theta_N,Psi_N,S,ztilde_k)
        H_constr=zeros(4,2*N);
        H_constr(1:4,1:2)=Hk;

        g_constr=zeros(size(H_constr,1),1);
        g_constr(1:4)=g;

        c1=H_constr*u-g_constr;

        q_u=Qu(1,1);
        Qu_hat=zeros(2*N,2*N);

        for k=3:2*N
            Qu_hat(k,k)=q_u;
        end

        c2=u'*Qu_hat*u-1;


        c3=u'*(Theta_N'*S*Theta_N)*u+2*ztilde_k'*Psi_N'*S*Theta_N*u-1+ztilde_k'*Psi_N'*S*Psi_N*ztilde_k;

        c=[c1;c2;c3];
        ceq=[];

        gradc=[H_constr' 2*Qu_hat*u 2*(Theta_N'*S*Theta_N)*u+(2*ztilde_k'*Psi_N'*S*Theta_N)'];
        gradceq=[];
    end


options=optimoptions('fmincon','Display','off','Algorithm','sqp-legacy','SpecifyObjectiveGradient',true,'SpecifyConstraintGradient',true);
[usol,fval,exitflag,output,lambda,grad,hessian] = fmincon(@(u)objective_function(u,H_obj,f_obj),zeros(N*2,1),[],[],[],[],[],[],@(u)quad_constr(u,Hk,g,Qu,N,Theta_N,Psi_N,S,ztilde_k),options);


viol=output.constrviolation;


uk=usol(1:2);



v=T_FL\uk;


end

== matlab function Trajectory_Tracking_Car_FL_MPC/Bycicle model  ==
  data: q input; qdot output; v1 input; v2 input; l input
function qdot  = bycicle_model(q,v1,v2,l)

%This function implements the car kinematic model
x=q(1);
y=q(2);
theta=q(3);
phi=q(4);

q1dot=v1*cos(theta);
q2dot=v1*sin(theta);
q3dot = v1*tan(phi)/l;
q4dot = v2;


qdot= [q1dot;q2dot;q3dot;q4dot];
end

== matlab function Trajectory_Tracking_Car_FL_MPC/Controller/MPC_fmincon ==
  data: q input; v output; qr input; vr input; l input; Delta input; N input; Ts input
function v = MPC_fmincon_tracking_controller(q,qr,vr,l,Delta,N,Ts)


qz=1; qu=0.1;


x=q(1); y=q(2); theta=q(3); phi=q(4);

%Feedback linearized system state
z_k=[x+l*cos(theta)+Delta*cos(phi+theta);
    y+l*sin(theta)+Delta*sin(phi+theta)];


Wr=zeros(2*N,1);
R=zeros(2*N,1);



for i=1:N
    xr=qr(1,i); yr=qr(2,i); thetar=qr(3,i); phir=qr(4,i);
    v1r=vr(1,i); v2r=vr(2,i);

    %Feedback linearized system reference at time k+i
    zr_k=[xr+l*cos(thetar)+Delta*cos(phir+thetar);
        yr+l*sin(thetar)+Delta*sin(phir+thetar)];

    R(2*i-1:2*i,1)=zr_k;

    %Feedback Linearization reference transformation
    T_FL_r=[cos(thetar)-tan(phir)*(sin(thetar)+Delta*sin(thetar+phir)/l) -Delta*sin(thetar+phir);
        sin(thetar)+tan(phir)*(cos(thetar)+Delta*cos(thetar+phir)/l) Delta*cos(thetar+phir)];

    ur_k=T_FL_r*[v1r;v2r];
    
    Wr(2*i-1:2*i,1)=ur_k;


end


Phi=repmat(eye(2),N,1);
Theta=Ts*repmat(eye(2),N);
Theta=tril(Theta);
Qhat=qz*eye(2*N);
Rhat=qu*eye(2*N);




T=[-1 0; 0 -1; 1 0; 0 1];
Hk=T/T_FL;
g=[v1max;v2max;v1max;v2max];




%Set theoretic MPC online optimization
obj_fun=@(W)(Phi*z_k+Theta*(W-Wr)-R)'*Qhat*(Phi*z_k+Theta*(W-Wr)-R)+W'*Rhat*W;


    function [c,ceq]=quad_constr(u,H,g,Qpre,ur,A,B,x_curr,Hk)
        c=Hk*(u+ur)-g;
        ceq=[];
        

        H_constr=zeros(4,2*N);
        H_constr(1:4,1:2)=Hk;

% for i=1:N-1
%     
%     H_constr(4+(i-1)*Nc+1:4+(i-1)*Nc+Nc,2*i+1:2*i+2)=H_w;
% 
% 
% end



g_constr=zeros(size(H_constr,1),1);
g_constr(1:4)=g;



    end



options=optimoptions('fmincon','Display','off','Algorithm','sqp');
usol = fmincon(obj_fun,zeros(N*2,1),[],[],[],[],[],[],[],options);
uk=usol(1:2);






%Feedback Linearization state transformation
T_FL=[cos(theta)-tan(phi)*(sin(theta)+Delta*sin(theta+phi)/l) -Delta*sin(theta+phi);
    sin(theta)+tan(phi)*(cos(theta)+Delta*cos(theta+phi)/l) Delta*cos(theta+phi)];



v=inv(T_FL)*uk;

== matlab function Trajectory_Tracking_Car_FL_MPC/Controller/MPC_active_set_original_conservative ==
  data: q input; v output; qr input; vr input; l input; Delta input; N input; Ts input; v1max input; v2max input; H_w input
function v = MPC_active_set_worst_case(q,qr,vr,l,Delta,N,Ts,v1max,v2max,H_w)


qz=1; qu=0.01;


x=q(1); y=q(2); theta=q(3); phi=q(4);

%Feedback linearized system state
z_k=[x+l*cos(theta)+Delta*cos(phi+theta);
    y+l*sin(theta)+Delta*sin(phi+theta)];


Wr=zeros(2*N,1);
R=zeros(2*N,1);



for i=1:N
    xr=qr(1,i); yr=qr(2,i); thetar=qr(3,i); phir=qr(4,i);
    v1r=vr(1,i); v2r=vr(2,i);

    %Feedback linearized system reference at time k+i
    zr_k=[xr+l*cos(thetar)+Delta*cos(phir+thetar);
        yr+l*sin(thetar)+Delta*sin(phir+thetar)];

    R(2*i-1:2*i,1)=zr_k;

    %Feedback Linearization reference transformation
    T_FL_r=[cos(thetar)-tan(phir)*(sin(thetar)+Delta*sin(thetar+phir)/l) -Delta*sin(thetar+phir);
        sin(thetar)+tan(phir)*(cos(thetar)+Delta*cos(thetar+phir)/l) Delta*cos(thetar+phir)];

    ur_k=T_FL_r*[v1r;v2r];

    Wr(2*i-1:2*i,1)=ur_k;


end


%Feedback Linearization state transformation
T_FL=[cos(theta)-tan(phi)*(sin(theta)+Delta*sin(theta+phi)/l) -Delta*sin(theta+phi);
    sin(theta)+tan(phi)*(cos(theta)+Delta*cos(theta+phi)/l) Delta*cos(theta+phi)];





Phi=repmat(eye(2),N,1);
Theta=Ts*repmat(eye(2),N);
Theta=tril(Theta);
Qhat=qz*eye(2*N);
Rhat=qu*eye(2*N);







H_obj=Theta'*Qhat*Theta+Rhat;
f_obj=Theta'*Qhat*Phi*z_k-Theta'*Qhat*Theta*Wr-Theta'*Qhat*R;

T=[-1 0; 0 -1; 1 0; 0 1];
Hk=T/T_FL;
g=[v1max;v2max;v1max;v2max];


Nc=size(H_w,1);
H_constr=zeros(4+Nc*(N-1),2*N);
H_constr(1:4,1:2)=Hk;

for i=1:N-1
    
    H_constr(4+(i-1)*Nc+1:4+(i-1)*Nc+Nc,2*i+1:2*i+2)=H_w;


end



g_constr=ones(size(H_constr,1),1);
g_constr(1:4)=g;




% options = optimoptions('quadprog','Algorithm','active-set');
% usol =  quadprog(H_obj,f_obj,H_constr,g_constr,[],[],[],[],zeros(2*N,1),options);




% opt.MaxIterations = 100;
% opt.ConstraintTolerance = 1.0e-6;
% opt.OptimalityTolerance = 1.0e-6;

opt = mpcInteriorPointOptions;
% usol=mpcInteriorPointSolver(H_obj,f_obj,H_constr,g_constr,zeros(0,2*N),zeros(0,1),zeros(2*N,1),opt);


opt.UseHessianAsInput = true;
iA0 = false(size(g_constr));
usol=mpcActiveSetSolver(H_obj,f_obj,H_constr,g_constr,zeros(0,2*N),zeros(0,1),iA0,opt);



uk=usol(1:2);



v=T_FL\uk;

== matlab function Trajectory_Tracking_Car_FL_MPC/Controller/MPC_active_set1 ==
  data: q input; v output; qr input; vr input; l input; Delta input; N input; Ts input; v1max input; v2max input
function v = MPC_active_set(q,qr,vr,l,Delta,N,Ts,v1max,v2max)


qz=1; qu=0.02;


x=q(1); y=q(2); theta=q(3); phi=q(4);

%Feedback linearized system state
z_k=[x+l*cos(theta)+Delta*cos(phi+theta);
    y+l*sin(theta)+Delta*sin(phi+theta)];


Wr=zeros(2*N,1);
R=zeros(2*N,1);



for i=1:N
    xr=qr(1,i); yr=qr(2,i); thetar=qr(3,i); phir=qr(4,i);
    v1r=vr(1,i); v2r=vr(2,i);

    %Feedback linearized system reference at time k+i
    zr_k=[xr+l*cos(thetar)+Delta*cos(phir+thetar);
        yr+l*sin(thetar)+Delta*sin(phir+thetar)];

    R(2*i-1:2*i,1)=zr_k;

    %Feedback Linearization reference transformation
    T_FL_r=[cos(thetar)-tan(phir)*(sin(thetar)+Delta*sin(thetar+phir)/l) -Delta*sin(thetar+phir);
        sin(thetar)+tan(phir)*(cos(thetar)+Delta*cos(thetar+phir)/l) Delta*cos(thetar+phir)];

    ur_k=T_FL_r*[v1r;v2r];

    Wr(2*i-1:2*i,1)=ur_k;


end


%Feedback Linearization state transformation
T_FL=[cos(theta)-tan(phi)*(sin(theta)+Delta*sin(theta+phi)/l) -Delta*sin(theta+phi);
    sin(theta)+tan(phi)*(cos(theta)+Delta*cos(theta+phi)/l) Delta*cos(theta+phi)];





Phi=repmat(eye(2),N,1);
Theta=Ts*repmat(eye(2),N);
Theta=tril(Theta);
Qhat=qz*eye(2*N);
Rhat=qu*eye(2*N);







H_obj=Theta'*Qhat*Theta+Rhat;
f_obj=Theta'*Qhat*Phi*z_k-Theta'*Qhat*Theta*Wr-Theta'*Qhat*R;

T=[-1 0; 0 -1; 1 0; 0 1];
Hk=T/T_FL;
g=[v1max;v2max;v1max;v2max];

H_constr=zeros(4*N,2*N);
H_constr(1:4,1:2)=Hk;

g_constr=zeros(4*N,1);
g_constr(1:4)=g;




% options = optimoptions('quadprog','Algorithm','active-set');
% usol =  quadprog(H_obj,f_obj,H_constr,g_constr,[],[],[],[],zeros(2*N,1),options);




% opt.MaxIterations = 100;
% opt.ConstraintTolerance = 1.0e-6;
% opt.OptimalityTolerance = 1.0e-6;

opt = mpcInteriorPointOptions;
% usol=mpcInteriorPointSolver(H_obj,f_obj,H_constr,g_constr,zeros(0,2*N),zeros(0,1),zeros(2*N,1),opt);


opt.UseHessianAsInput = true;
iA0 = false(size(g_constr));
usol=mpcActiveSetSolver(H_obj,f_obj,H_constr,g_constr,zeros(0,2*N),zeros(0,1),iA0,opt);



uk=usol(1:2);



v=T_FL\uk;
